simulink subsystem "cartesian_subsys"  (R2022b)
settings: Solver=VariableStepAuto  StartTime=0.0  StopTime=10.0  RelTol=1e-3
model mask{InitialCondition=0}
  mask prompts: InitialCondition "Simulink:blkprm_prompts:IntegratorInitCond"
libraries: dspsigops x1
settings Model: Creator=gotta  LastModifiedBy=giuliapegoraro

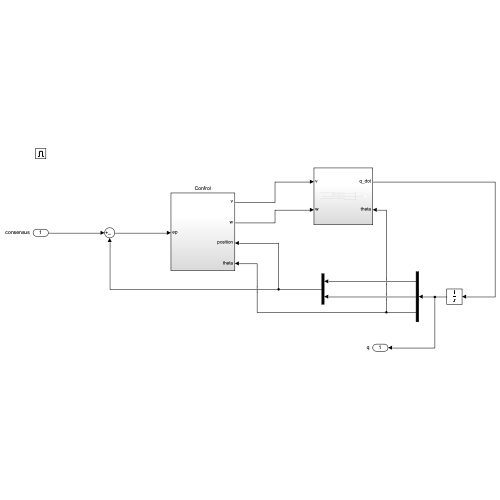
[thumbnail: Simulink's stored preview of the top-level diagram]
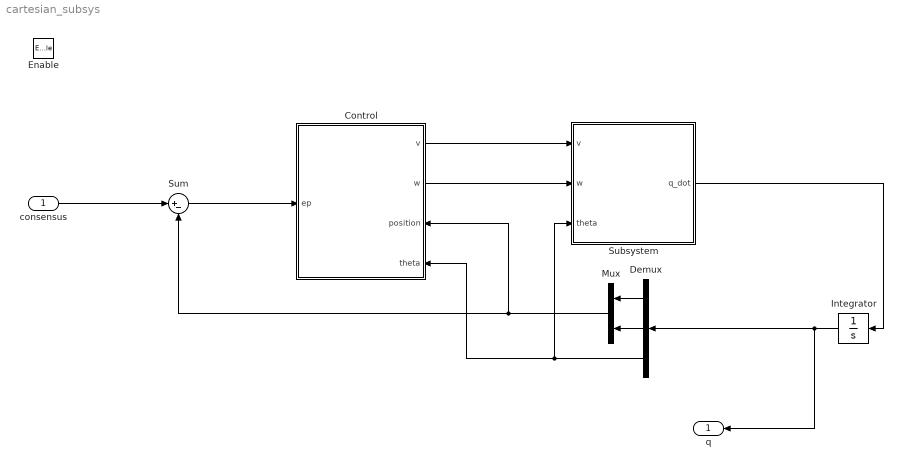
== system cartesian_subsys ==
  consensus : Inport
  Enable : EnablePort
  Control : Subsystem
      settings: PortSchema="{\"entries\":[{\"content\":{\"sides\":[{\"content\":{\"connectorIds\":[\"In1\"]},\"type\":\"ConnectorPlacement.EquallySpacedRectSide\",\"uuid\":\"d05dd044-a23a-4e4d-acf8-14e1672fb9ed\"},{\"content\":{\"connectorIds\":[\"Out1\",\"Out2\",\"In2\",\"In3\"],\"side\":\"RIGHT\"},\"type\":\"ConnectorPlacement.EquallySpacedRectSide\",\"uuid\":\"2fd26a19-9e2b-4967-a8eb-80a7dfa5e98f\"},{\"content\":{\"connectorIds\":[],\"side\":\"TOP\"},\"type\":\"ConnectorPlacement.EquallySpacedRectSide\",\"uuid\":\"c94760ad-869e-415a-9f16-9d32c94e7156\"}]},\"type\":\"ConnectorPlacement.EquallySpacedConnector\",\"uuid\":\"e7ddf13b-92e7-413e-b0f7-0c49af7708e3\"}],\"packageUris\":[\"http://schema.mathworks.com/mf0/Connector/R2020b\"],\"version\":\"1.0\"}"
  Demux : Demux  Outputs=3
  Integrator : Integrator  InitialCondition=InitialCondition
  Mux : Mux  Inputs=2
  Subsystem : Subsystem
  Sum : Sum  Inputs=|+-
  q : Outport
  wires:
  Demux/3 -> Subsystem/3(theta), Control/3(theta)
  Mux/1 -> Control/2(position), Sum/2
  Demux/2 -> Mux/2
  Demux/1 -> Mux/1
  Integrator/1 -> q/1, Demux/1
  Subsystem/1(q_dot) -> Integrator/1
  Control/2(w) -> Subsystem/2(w)
  Control/1(v) -> Subsystem/1(v)
  Sum/1 -> Control/1(ep)
  consensus/1 -> Sum/1

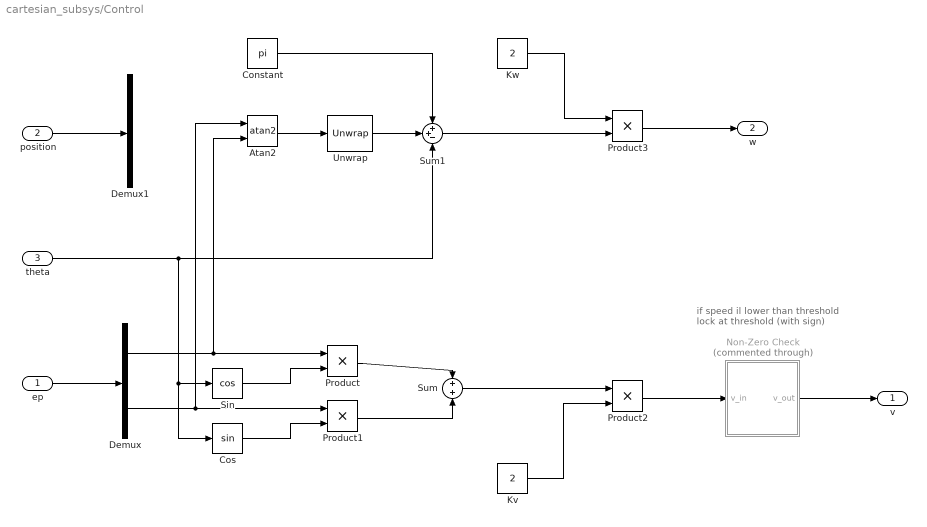
== system cartesian_subsys/Control ==
  note: if speed il lower than threshold
      | lock at threshold (with sign)
  ep : Inport
  position : Inport  Port=2
  theta : Inport  Port=3
  Atan2 : Trigonometry  Operator=atan2
  Constant : Constant  Value=pi
  Cos : Trigonometry
  Demux : Demux  Outputs=2
  Demux1 : Demux  Outputs=2
  Kv : Constant  Value=2
  Kw : Constant  Value=2
  Non-Zero Check : MATLAB Function  Commented=through  TreatAsAtomicUnit=on
  Product{,1..3} (4 alike) : Product
  Sin : Trigonometry  Operator=cos
  Sum : Sum  Inputs=+|+
  Sum1 : Sum  Inputs=++-
  Unwrap : dspsigops/Unwrap  tol=pi  InputProcessing=Columns as channels (frame based)  running=off
  v : Outport
  w : Outport  Port=2
  wires:
  Non-Zero Check/1(v_out) -> v/1
  Demux/2 -> Atan2/1, Product1/1
  Cos/1 -> Product1/2
  Demux/1 -> Atan2/2, Product/1
  Constant/1 -> Sum1/1
  Atan2/1 -> Unwrap/1
  position/1 -> Demux1/1
  ep/1 -> Demux/1
  theta/1 -> Sum1/3, Sin/1, Cos/1
  Sin/1 -> Product/2
  Product1/1 -> Sum/2
  Product/1 -> Sum/1
  Sum/1 -> Product2/1
  Kv/1 -> Product2/2
  Product2/1 -> Non-Zero Check/1(v_in)
  Sum1/1 -> Product3/2
  Kw/1 -> Product3/1
  Product3/1 -> w/1
  Unwrap/1 -> Sum1/2

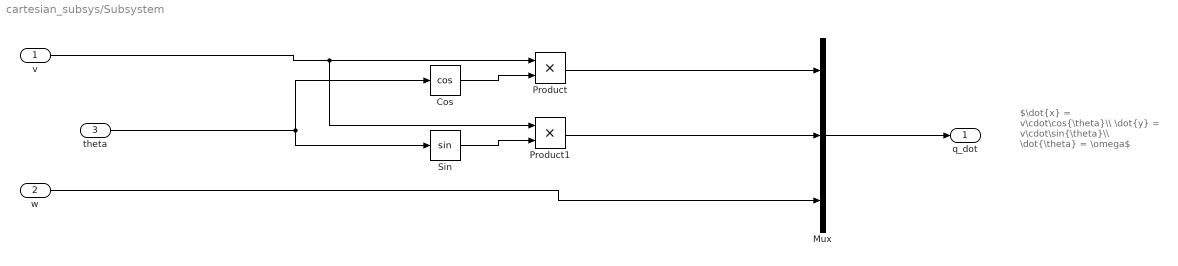
== system cartesian_subsys/Subsystem ==
  note: $\dot{x} = v\cdot\cos{\theta}\\ \dot{y} = v\cdot\sin{\theta}\\ \dot{\theta} = \omega$
  v : Inport
  w : Inport  Port=2
  theta : Inport  Port=3
  Cos : Trigonometry  Operator=cos
  Mux : Mux  Inputs=3
  Product : Product
  Product1 : Product
  Sin : Trigonometry
  q_dot : Outport
  wires:
  Sin/1 -> Product1/2
  v/1 -> Product/1, Product1/1
  w/1 -> Mux/3
  Cos/1 -> Product/2
  Mux/1 -> q_dot/1
  theta/1 -> Sin/1, Cos/1
  Product/1 -> Mux/1
  Product1/1 -> Mux/2

== matlab function cartesian_subsys/Control/Non-Zero Check ==
  data: v_in input; v_out output
function v_out = fcn(v_in)

if abs(v_in) < 1e-2
    if v_in >= 0 
        v_out = 1e-2;
    else 
        v_out = -1e-2;
    end
else
    v_out = v_in;
end
